simulink model "Stabilization_simulink"  (R2024b)
settings: Solver=ode4  StartTime=0.0  StopTime=1  FixedStep=1/200  RelTol=1e-3
values from neighbouring files (symbols this model uses):
  dz = 28*(pi/180)    (= 0.488692190558)    [Stabilization_Loop_Design.m]
  input_deg = 500    [Stabilization_Loop_Design.m]
  Ki = Wc^2 / Km    (= 29.520295203)    [Stabilization_Loop_Design.m]
  Km = 13.55    [Stabilization_Loop_Design.m]
  Kp = (2*Zc*Wc - Pm) / Km    (= 1.02878228782)    [Stabilization_Loop_Design.m]
  Pm = 14.06    [Stabilization_Loop_Design.m]
  W_sat = 1400    [Stabilization_Loop_Design.m]
  wb_dist = 10    [Stabilization_Loop_Design.m]
settings Model: Creator=chaeeun  LastModifiedBy=ADMIN
settings ConfigComp: CovBoundaryAbsTol=1.0e-5

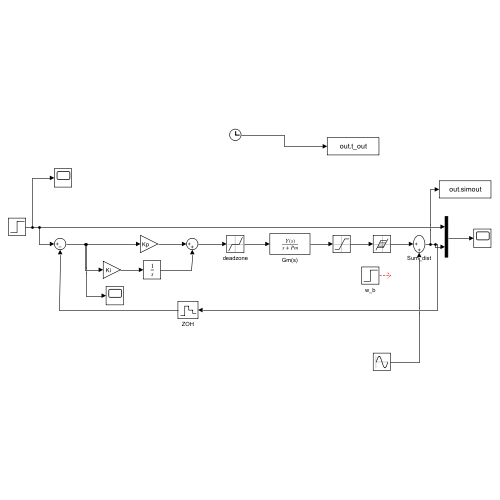
[thumbnail: Simulink's stored preview of the top-level diagram]
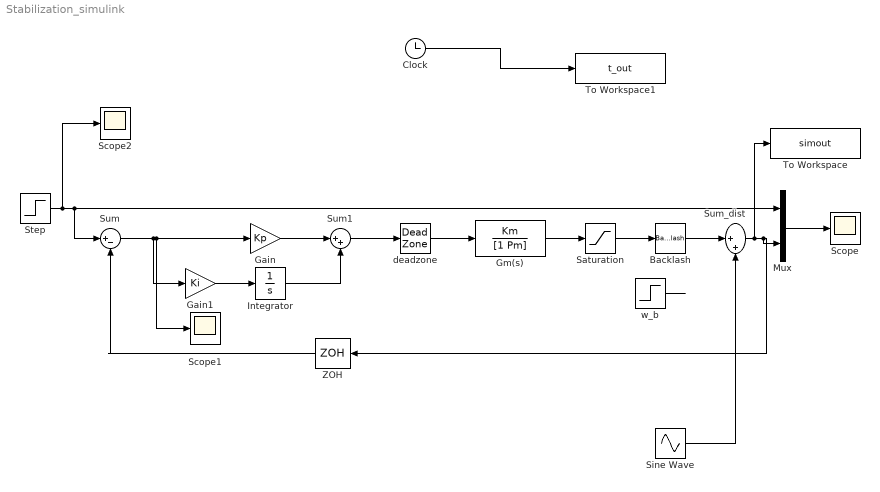
== system Stabilization_simulink ==
  Backlash : Backlash  BacklashWidth=0
  Clock : Clock
  Gain : Gain  Gain=Kp
  Gain1 : Gain  Gain=Ki
  Gm(s) : TransferFcn  Numerator=Km  Denominator=[1 Pm]
  Integrator : Integrator
  Mux : Mux  Inputs=2
  Saturation : Saturate  UpperLimit=W_sat  LowerLimit=-W_sat
  Scope : Scope
  Scope1 : Scope
  Scope2 : Scope
  Sine Wave : Sin  Frequency=0.5*2*pi  SampleTime=0
  Step : Step  Time=0  After=input_deg  SampleTime=0  VectorParams1D=off
  Sum : Sum  Inputs=|+-
  Sum1 : Sum  Inputs=|++
  Sum_dist : Sum  Inputs=|++
  To Workspace : ToWorkspace  VariableName=simout  SampleTime=0.005
      settings: Save2DSignal=2-D array (concatenate along first dimension)
  To Workspace1 : ToWorkspace  VariableName=t_out  SampleTime=0.005
      settings: Save2DSignal=2-D array (concatenate along first dimension)
  ZOH : ZeroOrderHold  SampleTime=1/200
  deadzone : DeadZone  LowerValue=-dz  UpperValue=dz
  w_b : Step  Time=0.25  After=wb_dist  SampleTime=0  VectorParams1D=off
  wires:
  ZOH/1 -> Sum/2
  Mux/1 -> Scope/1
  Step/1 -> Scope2/1, Mux/1, Sum/1
  Gain/1 -> Sum1/1
  Sum/1 -> Gain/1, Scope1/1, Gain1/1
  Gain1/1 -> Integrator/1
  Integrator/1 -> Sum1/2
  Sum1/1 -> deadzone/1
  deadzone/1 -> Gm(s)/1
  Gm(s)/1 -> Saturation/1
  Saturation/1 -> Backlash/1
  Backlash/1 -> Sum_dist/1
  w_b/1 -> ?
  Sine Wave/1 -> Sum_dist/2
  Sum_dist/1 -> ZOH/1, Mux/2, To Workspace/1
  Clock/1 -> To Workspace1/1
